simulink model "subsys_Events"  (Simulink 5.0)
settings: Solver=FixedStepDiscrete  StartTime=0.0  StopTime=10.0  RelTol=1e-3
settings Model: Creator=sofronis  LastModifiedBy=sofronis  ExtModeAutoUpdateStatusClock=off  AlgebraicLoopMsg=error

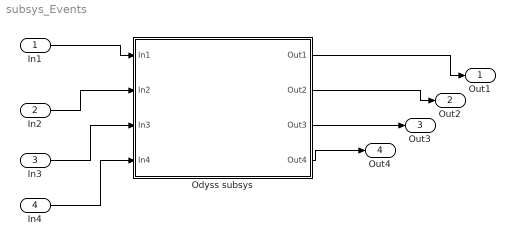
== system subsys_Events ==
  In1 : Inport  SampleTime=1
  In2 : Inport  Port=2  SampleTime=1
  In3 : Inport  Port=3  SampleTime=1
  In4 : Inport  Port=4  SampleTime=1
  Odyss subsys : Subsystem
  Out1 : Outport
  Out2 : Outport  Port=2
  Out3 : Outport  Port=3
  Out4 : Outport  Port=4
  wires:
  In1/1 -> Odyss subsys/1(In1)
  In2/1 -> Odyss subsys/2(In2)
  In3/1 -> Odyss subsys/3(In3)
  In4/1 -> Odyss subsys/4(In4)
  Odyss subsys/1(Out1) -> Out1/1
  Odyss subsys/2(Out2) -> Out2/1
  Odyss subsys/3(Out3) -> Out3/1
  Odyss subsys/4(Out4) -> Out4/1

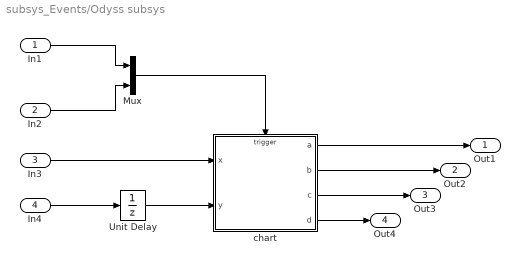
== system subsys_Events/Odyss subsys ==
  In1 : Inport  SampleTime=1
  In2 : Inport  Port=2  SampleTime=1
  In3 : Inport  Port=3  SampleTime=1
  In4 : Inport  Port=4  SampleTime=1
  Mux : Mux  Inputs=2
  Unit Delay : UnitDelay  SampleTime=-1
  chart : Stateflow chart
  Out1 : Outport
  Out2 : Outport  Port=2
  Out3 : Outport  Port=3
  Out4 : Outport  Port=4
  wires:
  In1/1 -> Mux/1
  In2/1 -> Mux/2
  In3/1 -> chart/1(x)
  Mux/1 -> chart/Trigger
  chart/1(a) -> Out1/1
  chart/2(b) -> Out2/1
  chart/3(c) -> Out3/1
  chart/4(d) -> Out4/1
  In4/1 -> Unit Delay/1
  Unit Delay/1 -> chart/2(y)

== stateflow chart Odyss subsys/chart ==
  state B [parallel]
    state Ba/
      en:b=x+3
    state Bb/
      en:b=x+4+y
    (default) -> Ba
    Bb -> Ba : R1/R2
    Ba -> Bb : S1/S2
  state A [parallel]
    state Aa/
      en:a=x+1
    state Ab/
      en:a=x+2
    (default) -> Aa
    Aa -> Ab : S/S1
    Ab -> Aa : R/R1
  state D [parallel]
    state Da/
      en:d=x+7
    state Db/
      en:d=x+8
    Db -> Da : R3
    (default) -> Da
    Da -> Db : S3
  state C [parallel]
    state Cb/
      en:c=x+6
    state Ca/
      en:c=x+5
    Ca -> Cb : S2/S3
    Cb -> Ca : R2/R3
    (default) -> Ca
  data: a output int32; x input int32; b output int32; c output int32; d output int32; y input int32
  events: R1 local EITHER_EDGE_EVENT; S1 local EITHER_EDGE_EVENT; R input RISING_EDGE_EVENT; S input FALLING_EDGE_EVENT; R2 local EITHER_EDGE_EVENT; S2 local EITHER_EDGE_EVENT; S3 local EITHER_EDGE_EVENT; R3 local EITHER_EDGE_EVENT
